simulink model "stereo_ibvs_core_backup_20260724_005942"  (R2025b)
settings: Solver=FixedStepDiscrete  StartTime=0.0  StopTime=10  FixedStep=cfg.Ts  RelTol=1e-3
InitFcn:
  | modelPath = get_param(bdroot,'FileName');
  |                                                                                       simulinkPath = fileparts(fileparts(modelPath));
  |                                                                                       configPath = fullfile(simulinkPath,'config','stereo_ibvs_config.m');
  |                                                                                       if ~isfile(configPath), error('StereoIBVS:ConfigNotFound','找不到配置文件：%s',configPath); end
  |                                                                                       run(configPath);
undefined symbols (not defined in the file): cfg
(part 2 of 4)

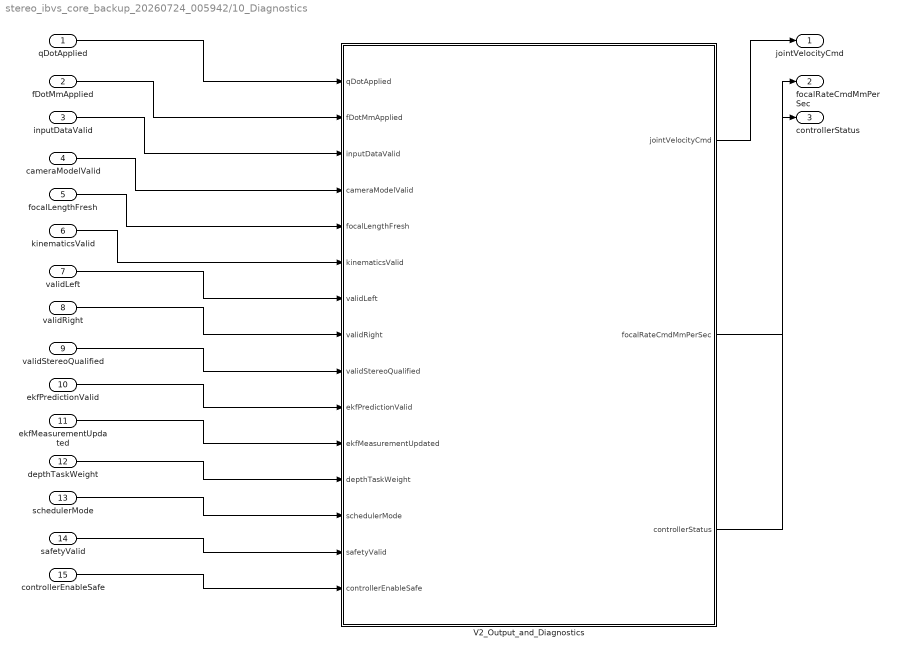
== system stereo_ibvs_core_backup_20260724_005942/10_Diagnostics ==
  qDotApplied : Inport  OutDataTypeStr=double  PortDimensions=[7 1]
  fDotMmApplied : Inport  Port=2  OutDataTypeStr=double  PortDimensions=[2 1]
  inputDataValid : Inport  Port=3  OutDataTypeStr=double  PortDimensions=1
  cameraModelValid : Inport  Port=4  OutDataTypeStr=double  PortDimensions=1
  focalLengthFresh : Inport  Port=5  OutDataTypeStr=double  PortDimensions=1
  kinematicsValid : Inport  Port=6  OutDataTypeStr=double  PortDimensions=1
  validLeft : Inport  Port=7  OutDataTypeStr=double  PortDimensions=1
  validRight : Inport  Port=8  OutDataTypeStr=double  PortDimensions=1
  validStereoQualified : Inport  Port=9  OutDataTypeStr=double  PortDimensions=1
  ekfPredictionValid : Inport  Port=10  OutDataTypeStr=double  PortDimensions=1
  ekfMeasurementUpdated : Inport  Port=11  OutDataTypeStr=double  PortDimensions=1
  depthTaskWeight : Inport  Port=12  OutDataTypeStr=double  PortDimensions=1
  schedulerMode : Inport  Port=13  OutDataTypeStr=double  PortDimensions=1
  safetyValid : Inport  Port=14  OutDataTypeStr=double  PortDimensions=1
  controllerEnableSafe : Inport  Port=15  OutDataTypeStr=double  PortDimensions=1
  V2_Output_and_Diagnostics : MATLAB Function  TreatAsAtomicUnit=on
  jointVelocityCmd : Outport  PortDimensions=[7 1]
  focalRateCmdMmPerSec : Outport  Port=2  PortDimensions=[2 1]
  controllerStatus : Outport  Port=3  PortDimensions=[13 1]
  wires:
  ? -> ?
  qDotApplied/1 -> V2_Output_and_Diagnostics/1(qDotApplied)
  fDotMmApplied/1 -> V2_Output_and_Diagnostics/2(fDotMmApplied)
  inputDataValid/1 -> V2_Output_and_Diagnostics/3(inputDataValid)
  cameraModelValid/1 -> V2_Output_and_Diagnostics/4(cameraModelValid)
  focalLengthFresh/1 -> V2_Output_and_Diagnostics/5(focalLengthFresh)
  kinematicsValid/1 -> V2_Output_and_Diagnostics/6(kinematicsValid)
  validLeft/1 -> V2_Output_and_Diagnostics/7(validLeft)
  validRight/1 -> V2_Output_and_Diagnostics/8(validRight)
  validStereoQualified/1 -> V2_Output_and_Diagnostics/9(validStereoQualified)
  ekfPredictionValid/1 -> V2_Output_and_Diagnostics/10(ekfPredictionValid)
  ekfMeasurementUpdated/1 -> V2_Output_and_Diagnostics/11(ekfMeasurementUpdated)
  depthTaskWeight/1 -> V2_Output_and_Diagnostics/12(depthTaskWeight)
  schedulerMode/1 -> V2_Output_and_Diagnostics/13(schedulerMode)
  safetyValid/1 -> V2_Output_and_Diagnostics/14(safetyValid)
  controllerEnableSafe/1 -> V2_Output_and_Diagnostics/15(controllerEnableSafe)
  V2_Output_and_Diagnostics/1(jointVelocityCmd) -> jointVelocityCmd/1
  V2_Output_and_Diagnostics/2(focalRateCmdMmPerSec) -> focalRateCmdMmPerSec/1
  V2_Output_and_Diagnostics/3(controllerStatus) -> controllerStatus/1

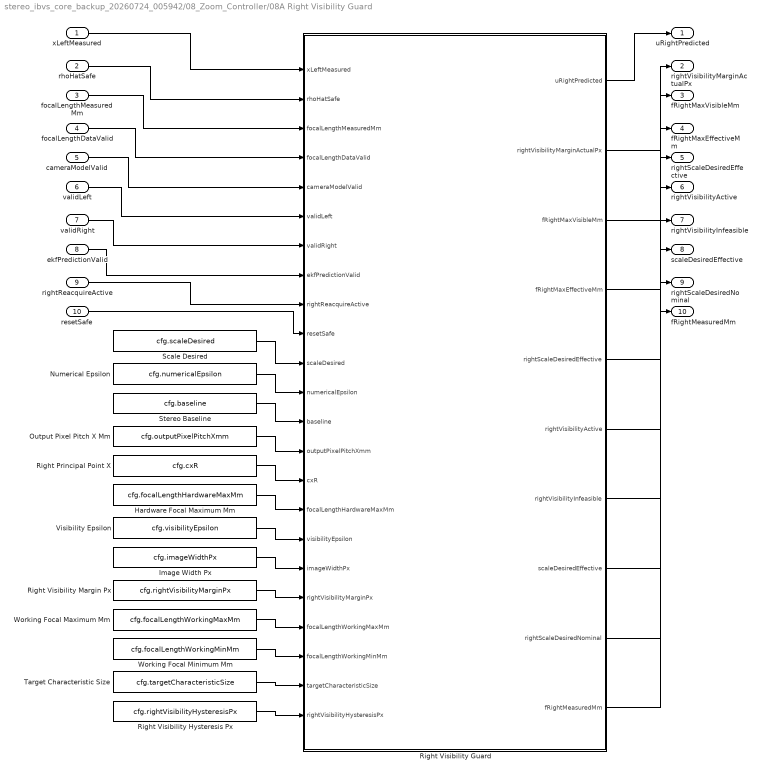
== system stereo_ibvs_core_backup_20260724_005942/08_Zoom_Controller/08A Right Visibility Guard ==
  xLeftMeasured : Inport  OutDataTypeStr=double  PortDimensions=1
  rhoHatSafe : Inport  Port=2  OutDataTypeStr=double  PortDimensions=1
  focalLengthMeasuredMm : Inport  Port=3  OutDataTypeStr=double  PortDimensions=[2 1]
  focalLengthDataValid : Inport  Port=4  OutDataTypeStr=double  PortDimensions=1
  cameraModelValid : Inport  Port=5  OutDataTypeStr=double  PortDimensions=1
  validLeft : Inport  Port=6  OutDataTypeStr=double  PortDimensions=1
  validRight : Inport  Port=7  OutDataTypeStr=double  PortDimensions=1
  ekfPredictionValid : Inport  Port=8  OutDataTypeStr=double  PortDimensions=1
  rightReacquireActive : Inport  Port=9  OutDataTypeStr=double  PortDimensions=1
  resetSafe : Inport  Port=10  OutDataTypeStr=double  PortDimensions=1
  Hardware Focal Maximum Mm : Constant  Value=cfg.focalLengthHardwareMaxMm  OutDataTypeStr=double  SampleTime=-1
  Image Width Px : Constant  Value=cfg.imageWidthPx  OutDataTypeStr=double  SampleTime=-1
  Numerical Epsilon : Constant  Value=cfg.numericalEpsilon  OutDataTypeStr=double  SampleTime=-1
  Output Pixel Pitch X Mm : Constant  Value=cfg.outputPixelPitchXmm  OutDataTypeStr=double  SampleTime=-1
  Right Principal Point X : Constant  Value=cfg.cxR  OutDataTypeStr=double  SampleTime=-1
  Right Visibility Guard : MATLAB Function  TreatAsAtomicUnit=on
  Right Visibility Hysteresis Px : Constant  Value=cfg.rightVisibilityHysteresisPx  OutDataTypeStr=double  SampleTime=-1
  Right Visibility Margin Px : Constant  Value=cfg.rightVisibilityMarginPx  OutDataTypeStr=double  SampleTime=-1
  Scale Desired : Constant  Value=cfg.scaleDesired  OutDataTypeStr=double  SampleTime=-1
  Stereo Baseline : Constant  Value=cfg.baseline  OutDataTypeStr=double  SampleTime=-1
  Target Characteristic Size : Constant  Value=cfg.targetCharacteristicSize  OutDataTypeStr=double  SampleTime=-1
  Visibility Epsilon : Constant  Value=cfg.visibilityEpsilon  OutDataTypeStr=double  SampleTime=-1
  Working Focal Maximum Mm : Constant  Value=cfg.focalLengthWorkingMaxMm  OutDataTypeStr=double  SampleTime=-1
  Working Focal Minimum Mm : Constant  Value=cfg.focalLengthWorkingMinMm  OutDataTypeStr=double  SampleTime=-1
  uRightPredicted : Outport  PortDimensions=1
  rightVisibilityMarginActualPx : Outport  Port=2  PortDimensions=1
  fRightMaxVisibleMm : Outport  Port=3  PortDimensions=1
  fRightMaxEffectiveMm : Outport  Port=4  PortDimensions=1
  rightScaleDesiredEffective : Outport  Port=5  PortDimensions=1
  rightVisibilityActive : Outport  Port=6  PortDimensions=1
  rightVisibilityInfeasible : Outport  Port=7  PortDimensions=1
  scaleDesiredEffective : Outport  Port=8  PortDimensions=[2 1]
  rightScaleDesiredNominal : Outport  Port=9  PortDimensions=1
  fRightMeasuredMm : Outport  Port=10  PortDimensions=1
  wires:
  ? -> ?
  xLeftMeasured/1 -> Right Visibility Guard/1(xLeftMeasured)
  rhoHatSafe/1 -> Right Visibility Guard/2(rhoHatSafe)
  focalLengthMeasuredMm/1 -> Right Visibility Guard/3(focalLengthMeasuredMm)
  focalLengthDataValid/1 -> Right Visibility Guard/4(focalLengthDataValid)
  cameraModelValid/1 -> Right Visibility Guard/5(cameraModelValid)
  validLeft/1 -> Right Visibility Guard/6(validLeft)
  validRight/1 -> Right Visibility Guard/7(validRight)
  ekfPredictionValid/1 -> Right Visibility Guard/8(ekfPredictionValid)
  rightReacquireActive/1 -> Right Visibility Guard/9(rightReacquireActive)
  resetSafe/1 -> Right Visibility Guard/10(resetSafe)
  Scale Desired/1 -> Right Visibility Guard/11(scaleDesired)
  Numerical Epsilon/1 -> Right Visibility Guard/12(numericalEpsilon)
  Stereo Baseline/1 -> Right Visibility Guard/13(baseline)
  Output Pixel Pitch X Mm/1 -> Right Visibility Guard/14(outputPixelPitchXmm)
  Right Principal Point X/1 -> Right Visibility Guard/15(cxR)
  Hardware Focal Maximum Mm/1 -> Right Visibility Guard/16(focalLengthHardwareMaxMm)
  Visibility Epsilon/1 -> Right Visibility Guard/17(visibilityEpsilon)
  Image Width Px/1 -> Right Visibility Guard/18(imageWidthPx)
  Right Visibility Margin Px/1 -> Right Visibility Guard/19(rightVisibilityMarginPx)
  Working Focal Maximum Mm/1 -> Right Visibility Guard/20(focalLengthWorkingMaxMm)
  Working Focal Minimum Mm/1 -> Right Visibility Guard/21(focalLengthWorkingMinMm)
  Target Characteristic Size/1 -> Right Visibility Guard/22(targetCharacteristicSize)
  Right Visibility Hysteresis Px/1 -> Right Visibility Guard/23(rightVisibilityHysteresisPx)
  Right Visibility Guard/1(uRightPredicted) -> uRightPredicted/1
  Right Visibility Guard/2(rightVisibilityMarginActualPx) -> rightVisibilityMarginActualPx/1
  Right Visibility Guard/3(fRightMaxVisibleMm) -> fRightMaxVisibleMm/1
  Right Visibility Guard/4(fRightMaxEffectiveMm) -> fRightMaxEffectiveMm/1
  Right Visibility Guard/5(rightScaleDesiredEffective) -> rightScaleDesiredEffective/1
  Right Visibility Guard/6(rightVisibilityActive) -> rightVisibilityActive/1
  Right Visibility Guard/7(rightVisibilityInfeasible) -> rightVisibilityInfeasible/1
  Right Visibility Guard/8(scaleDesiredEffective) -> scaleDesiredEffective/1
  Right Visibility Guard/9(rightScaleDesiredNominal) -> rightScaleDesiredNominal/1
  Right Visibility Guard/10(fRightMeasuredMm) -> fRightMeasuredMm/1

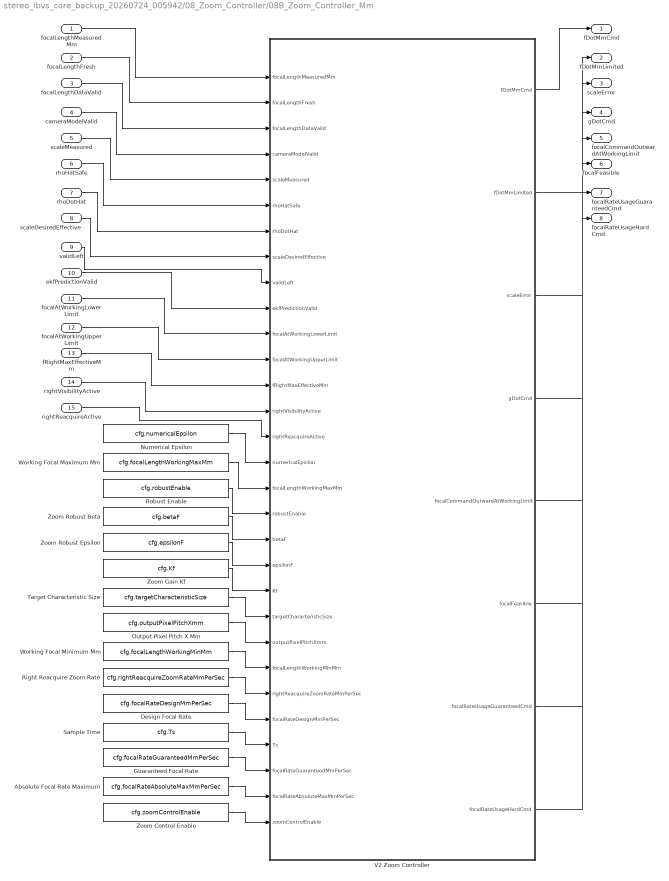
== system stereo_ibvs_core_backup_20260724_005942/08_Zoom_Controller/08B_Zoom_Controller_Mm ==
  focalLengthMeasuredMm : Inport  OutDataTypeStr=double  PortDimensions=[2 1]
  focalLengthFresh : Inport  Port=2  OutDataTypeStr=double  PortDimensions=1
  focalLengthDataValid : Inport  Port=3  OutDataTypeStr=double  PortDimensions=1
  cameraModelValid : Inport  Port=4  OutDataTypeStr=double  PortDimensions=1
  scaleMeasured : Inport  Port=5  OutDataTypeStr=double  PortDimensions=[2 1]
  rhoHatSafe : Inport  Port=6  OutDataTypeStr=double  PortDimensions=1
  rhoDotHat : Inport  Port=7  OutDataTypeStr=double  PortDimensions=[2 1]
  scaleDesiredEffective : Inport  Port=8  OutDataTypeStr=double  PortDimensions=[2 1]
  validLeft : Inport  Port=9  OutDataTypeStr=double  PortDimensions=1
  ekfPredictionValid : Inport  Port=10  OutDataTypeStr=double  PortDimensions=1
  focalAtWorkingLowerLimit : Inport  Port=11  OutDataTypeStr=double  PortDimensions=[2 1]
  focalAtWorkingUpperLimit : Inport  Port=12  OutDataTypeStr=double  PortDimensions=[2 1]
  fRightMaxEffectiveMm : Inport  Port=13  OutDataTypeStr=double  PortDimensions=1
  rightVisibilityActive : Inport  Port=14  OutDataTypeStr=double  PortDimensions=1
  rightReacquireActive : Inport  Port=15  OutDataTypeStr=double  PortDimensions=1
  Absolute Focal Rate Maximum : Constant  Value=cfg.focalRateAbsoluteMaxMmPerSec  OutDataTypeStr=double  SampleTime=-1
  Design Focal Rate : Constant  Value=cfg.focalRateDesignMmPerSec  OutDataTypeStr=double  SampleTime=-1
  Guaranteed Focal Rate : Constant  Value=cfg.focalRateGuaranteedMmPerSec  OutDataTypeStr=double  SampleTime=-1
  Numerical Epsilon : Constant  Value=cfg.numericalEpsilon  OutDataTypeStr=double  SampleTime=-1
  Output Pixel Pitch X Mm : Constant  Value=cfg.outputPixelPitchXmm  OutDataTypeStr=double  SampleTime=-1
  Right Reacquire Zoom Rate : Constant  Value=cfg.rightReacquireZoomRateMmPerSec  OutDataTypeStr=double  SampleTime=-1
  Robust Enable : Constant  Value=cfg.robustEnable  OutDataTypeStr=double  SampleTime=-1
  Sample Time : Constant  Value=cfg.Ts  OutDataTypeStr=double  SampleTime=-1
  Target Characteristic Size : Constant  Value=cfg.targetCharacteristicSize  OutDataTypeStr=double  SampleTime=-1
  V2 Zoom Controller : MATLAB Function  TreatAsAtomicUnit=on
  Working Focal Maximum Mm : Constant  Value=cfg.focalLengthWorkingMaxMm  OutDataTypeStr=double  SampleTime=-1
  Working Focal Minimum Mm : Constant  Value=cfg.focalLengthWorkingMinMm  OutDataTypeStr=double  SampleTime=-1
  Zoom Control Enable : Constant  Value=cfg.zoomControlEnable  OutDataTypeStr=double  SampleTime=-1
  Zoom Gain Kf : Constant  Value=cfg.Kf  OutDataTypeStr=double  SampleTime=-1
  Zoom Robust Beta : Constant  Value=cfg.betaF  OutDataTypeStr=double  SampleTime=-1
  Zoom Robust Epsilon : Constant  Value=cfg.epsilonF  OutDataTypeStr=double  SampleTime=-1
  fDotMmCmd : Outport  PortDimensions=[2 1]
  fDotMmLimited : Outport  Port=2  PortDimensions=[2 1]
  scaleError : Outport  Port=3  PortDimensions=[2 1]
  gDotCmd : Outport  Port=4  PortDimensions=[2 1]
  focalCommandOutwardAtWorkingLimit : Outport  Port=5  PortDimensions=[2 1]
  focalFeasible : Outport  Port=6  PortDimensions=[2 1]
  focalRateUsageGuaranteedCmd : Outport  Port=7  PortDimensions=[2 1]
  focalRateUsageHardCmd : Outport  Port=8  PortDimensions=[2 1]
  wires:
  ? -> ?
  focalLengthMeasuredMm/1 -> V2 Zoom Controller/1(focalLengthMeasuredMm)
  focalLengthFresh/1 -> V2 Zoom Controller/2(focalLengthFresh)
  focalLengthDataValid/1 -> V2 Zoom Controller/3(focalLengthDataValid)
  cameraModelValid/1 -> V2 Zoom Controller/4(cameraModelValid)
  scaleMeasured/1 -> V2 Zoom Controller/5(scaleMeasured)
  rhoHatSafe/1 -> V2 Zoom Controller/6(rhoHatSafe)
  rhoDotHat/1 -> V2 Zoom Controller/7(rhoDotHat)
  scaleDesiredEffective/1 -> V2 Zoom Controller/8(scaleDesiredEffective)
  validLeft/1 -> V2 Zoom Controller/9(validLeft)
  ekfPredictionValid/1 -> V2 Zoom Controller/10(ekfPredictionValid)
  focalAtWorkingLowerLimit/1 -> V2 Zoom Controller/11(focalAtWorkingLowerLimit)
  focalAtWorkingUpperLimit/1 -> V2 Zoom Controller/12(focalAtWorkingUpperLimit)
  fRightMaxEffectiveMm/1 -> V2 Zoom Controller/13(fRightMaxEffectiveMm)
  rightVisibilityActive/1 -> V2 Zoom Controller/14(rightVisibilityActive)
  rightReacquireActive/1 -> V2 Zoom Controller/15(rightReacquireActive)
  Numerical Epsilon/1 -> V2 Zoom Controller/16(numericalEpsilon)
  Working Focal Maximum Mm/1 -> V2 Zoom Controller/17(focalLengthWorkingMaxMm)
  Robust Enable/1 -> V2 Zoom Controller/18(robustEnable)
  Zoom Robust Beta/1 -> V2 Zoom Controller/19(betaF)
  Zoom Robust Epsilon/1 -> V2 Zoom Controller/20(epsilonF)
  Zoom Gain Kf/1 -> V2 Zoom Controller/21(Kf)
  Target Characteristic Size/1 -> V2 Zoom Controller/22(targetCharacteristicSize)
  Output Pixel Pitch X Mm/1 -> V2 Zoom Controller/23(outputPixelPitchXmm)
  Working Focal Minimum Mm/1 -> V2 Zoom Controller/24(focalLengthWorkingMinMm)
  Right Reacquire Zoom Rate/1 -> V2 Zoom Controller/25(rightReacquireZoomRateMmPerSec)
  Design Focal Rate/1 -> V2 Zoom Controller/26(focalRateDesignMmPerSec)
  Sample Time/1 -> V2 Zoom Controller/27(Ts)
  Guaranteed Focal Rate/1 -> V2 Zoom Controller/28(focalRateGuaranteedMmPerSec)
  Absolute Focal Rate Maximum/1 -> V2 Zoom Controller/29(focalRateAbsoluteMaxMmPerSec)
  Zoom Control Enable/1 -> V2 Zoom Controller/30(zoomControlEnable)
  V2 Zoom Controller/1(fDotMmCmd) -> fDotMmCmd/1
  V2 Zoom Controller/2(fDotMmLimited) -> fDotMmLimited/1
  V2 Zoom Controller/3(scaleError) -> scaleError/1
  V2 Zoom Controller/4(gDotCmd) -> gDotCmd/1
  V2 Zoom Controller/5(focalCommandOutwardAtWorkingLimit) -> focalCommandOutwardAtWorkingLimit/1
  V2 Zoom Controller/6(focalFeasible) -> focalFeasible/1
  V2 Zoom Controller/7(focalRateUsageGuaranteedCmd) -> focalRateUsageGuaranteedCmd/1
  V2 Zoom Controller/8(focalRateUsageHardCmd) -> focalRateUsageHardCmd/1

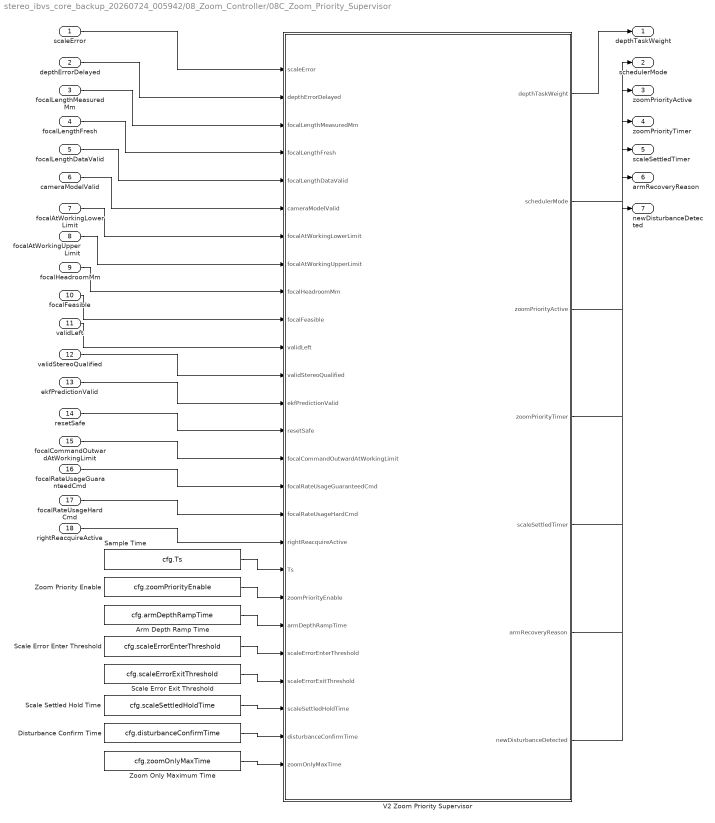
== system stereo_ibvs_core_backup_20260724_005942/08_Zoom_Controller/08C_Zoom_Priority_Supervisor ==
  scaleError : Inport  OutDataTypeStr=double  PortDimensions=[2 1]
  depthErrorDelayed : Inport  Port=2  OutDataTypeStr=double  PortDimensions=1
  focalLengthMeasuredMm : Inport  Port=3  OutDataTypeStr=double  PortDimensions=[2 1]
  focalLengthFresh : Inport  Port=4  OutDataTypeStr=double  PortDimensions=1
  focalLengthDataValid : Inport  Port=5  OutDataTypeStr=double  PortDimensions=1
  cameraModelValid : Inport  Port=6  OutDataTypeStr=double  PortDimensions=1
  focalAtWorkingLowerLimit : Inport  Port=7  OutDataTypeStr=double  PortDimensions=[2 1]
  focalAtWorkingUpperLimit : Inport  Port=8  OutDataTypeStr=double  PortDimensions=[2 1]
  focalHeadroomMm : Inport  Port=9  OutDataTypeStr=double  PortDimensions=[2 1]
  focalFeasible : Inport  Port=10  OutDataTypeStr=double  PortDimensions=[2 1]
  validLeft : Inport  Port=11  OutDataTypeStr=double  PortDimensions=1
  validStereoQualified : Inport  Port=12  OutDataTypeStr=double  PortDimensions=1
  ekfPredictionValid : Inport  Port=13  OutDataTypeStr=double  PortDimensions=1
  resetSafe : Inport  Port=14  OutDataTypeStr=double  PortDimensions=1
  focalCommandOutwardAtWorkingLimit : Inport  Port=15  OutDataTypeStr=double  PortDimensions=[2 1]
  focalRateUsageGuaranteedCmd : Inport  Port=16  OutDataTypeStr=double  PortDimensions=[2 1]
  focalRateUsageHardCmd : Inport  Port=17  OutDataTypeStr=double  PortDimensions=[2 1]
  rightReacquireActive : Inport  Port=18  OutDataTypeStr=double  PortDimensions=1
  Arm Depth Ramp Time : Constant  Value=cfg.armDepthRampTime  OutDataTypeStr=double  SampleTime=-1
  Disturbance Confirm Time : Constant  Value=cfg.disturbanceConfirmTime  OutDataTypeStr=double  SampleTime=-1
  Sample Time : Constant  Value=cfg.Ts  OutDataTypeStr=double  SampleTime=-1
  Scale Error Enter Threshold : Constant  Value=cfg.scaleErrorEnterThreshold  OutDataTypeStr=double  SampleTime=-1
  Scale Error Exit Threshold : Constant  Value=cfg.scaleErrorExitThreshold  OutDataTypeStr=double  SampleTime=-1
  Scale Settled Hold Time : Constant  Value=cfg.scaleSettledHoldTime  OutDataTypeStr=double  SampleTime=-1
  V2 Zoom Priority Supervisor : MATLAB Function  TreatAsAtomicUnit=on
  Zoom Only Maximum Time : Constant  Value=cfg.zoomOnlyMaxTime  OutDataTypeStr=double  SampleTime=-1
  Zoom Priority Enable : Constant  Value=cfg.zoomPriorityEnable  OutDataTypeStr=double  SampleTime=-1
  depthTaskWeight : Outport  PortDimensions=1
  schedulerMode : Outport  Port=2  PortDimensions=1
  zoomPriorityActive : Outport  Port=3  PortDimensions=1
  zoomPriorityTimer : Outport  Port=4  PortDimensions=1
  scaleSettledTimer : Outport  Port=5  PortDimensions=1
  armRecoveryReason : Outport  Port=6  PortDimensions=1
  newDisturbanceDetected : Outport  Port=7  PortDimensions=1
  wires:
  ? -> ?
  scaleError/1 -> V2 Zoom Priority Supervisor/1(scaleError)
  depthErrorDelayed/1 -> V2 Zoom Priority Supervisor/2(depthErrorDelayed)
  focalLengthMeasuredMm/1 -> V2 Zoom Priority Supervisor/3(focalLengthMeasuredMm)
  focalLengthFresh/1 -> V2 Zoom Priority Supervisor/4(focalLengthFresh)
  focalLengthDataValid/1 -> V2 Zoom Priority Supervisor/5(focalLengthDataValid)
  cameraModelValid/1 -> V2 Zoom Priority Supervisor/6(cameraModelValid)
  focalAtWorkingLowerLimit/1 -> V2 Zoom Priority Supervisor/7(focalAtWorkingLowerLimit)
  focalAtWorkingUpperLimit/1 -> V2 Zoom Priority Supervisor/8(focalAtWorkingUpperLimit)
  focalHeadroomMm/1 -> V2 Zoom Priority Supervisor/9(focalHeadroomMm)
  focalFeasible/1 -> V2 Zoom Priority Supervisor/10(focalFeasible)
  validLeft/1 -> V2 Zoom Priority Supervisor/11(validLeft)
  validStereoQualified/1 -> V2 Zoom Priority Supervisor/12(validStereoQualified)
  ekfPredictionValid/1 -> V2 Zoom Priority Supervisor/13(ekfPredictionValid)
  resetSafe/1 -> V2 Zoom Priority Supervisor/14(resetSafe)
  focalCommandOutwardAtWorkingLimit/1 -> V2 Zoom Priority Supervisor/15(focalCommandOutwardAtWorkingLimit)
  focalRateUsageGuaranteedCmd/1 -> V2 Zoom Priority Supervisor/16(focalRateUsageGuaranteedCmd)
  focalRateUsageHardCmd/1 -> V2 Zoom Priority Supervisor/17(focalRateUsageHardCmd)
  rightReacquireActive/1 -> V2 Zoom Priority Supervisor/18(rightReacquireActive)
  Sample Time/1 -> V2 Zoom Priority Supervisor/19(Ts)
  Zoom Priority Enable/1 -> V2 Zoom Priority Supervisor/20(zoomPriorityEnable)
  Arm Depth Ramp Time/1 -> V2 Zoom Priority Supervisor/21(armDepthRampTime)
  Scale Error Enter Threshold/1 -> V2 Zoom Priority Supervisor/22(scaleErrorEnterThreshold)
  Scale Error Exit Threshold/1 -> V2 Zoom Priority Supervisor/23(scaleErrorExitThreshold)
  Scale Settled Hold Time/1 -> V2 Zoom Priority Supervisor/24(scaleSettledHoldTime)
  Disturbance Confirm Time/1 -> V2 Zoom Priority Supervisor/25(disturbanceConfirmTime)
  Zoom Only Maximum Time/1 -> V2 Zoom Priority Supervisor/26(zoomOnlyMaxTime)
  V2 Zoom Priority Supervisor/1(depthTaskWeight) -> depthTaskWeight/1
  V2 Zoom Priority Supervisor/2(schedulerMode) -> schedulerMode/1
  V2 Zoom Priority Supervisor/3(zoomPriorityActive) -> zoomPriorityActive/1
  V2 Zoom Priority Supervisor/4(zoomPriorityTimer) -> zoomPriorityTimer/1
  V2 Zoom Priority Supervisor/5(scaleSettledTimer) -> scaleSettledTimer/1
  V2 Zoom Priority Supervisor/6(armRecoveryReason) -> armRecoveryReason/1
  V2 Zoom Priority Supervisor/7(newDisturbanceDetected) -> newDisturbanceDetected/1

== matlab function stereo_ibvs_core_backup_20260724_005942/03_Feature_Processing/Normalize and Validate Features ==
  data: pixelMeasurement input; normalizedFeatureMeasured output; scaleMeasuredRaw input; fxMeasuredPx input; fyMeasuredPx input; validLeft input; validRight input; visionMeasurementNew input; resetSafe input; cfg_numericalEpsilon input; cfg_cxL input; cfg_cyL input; cfg_cxR input; cfg_cyR input; cfg_baseline input; cfg_disparityMin input; cfg_rhoMin input; cfg_rhoMax input; cfg_rightReacquireValidSamples input; cLMeasured output; cRMeasured output; scaleMeasured output; zMeasured output; xLeftMeasured output; yLeftMeasured output; xRightMeasured output; disparityNormalized output; rhoMeasured output; validDisparity output; stereoMeasurementEnable output; validStereoQualified output; rightReacquireActive output; rightReacquireCount output; uRightMeasured output
function [ ...
    normalizedFeatureMeasured, ...
    cLMeasured, ...
    cRMeasured, ...
    scaleMeasured, ...
    zMeasured, ...
    xLeftMeasured, ...
    yLeftMeasured, ...
    xRightMeasured, ...
    disparityNormalized, ...
    rhoMeasured, ...
    validDisparity, ...
    stereoMeasurementEnable, ...
    validStereoQualified, ...
    rightReacquireActive, ...
    rightReacquireCount, ...
    uRightMeasured] = fcn( ...
    pixelMeasurement, ...
    scaleMeasuredRaw, ...
    fxMeasuredPx, ...
    fyMeasuredPx, ...
    validLeft, ...
    validRight, ...
    visionMeasurementNew, ...
    resetSafe, ...
    cfg_numericalEpsilon, ...
    cfg_cxL, ...
    cfg_cyL, ...
    cfg_cxR, ...
    cfg_cyR, ...
    cfg_baseline, ...
    cfg_disparityMin, ...
    cfg_rhoMin, ...
    cfg_rhoMax, ...
    cfg_rightReacquireValidSamples)
%#codegen
% V2实机视觉测量提取与双目有效性管理。
% cfg_* 均由外部 Constant 块输入，不再登记为 MATLAB Function Parameter。

%% 固定尺寸输出
normalizedFeatureMeasured = zeros(4,1);
cLMeasured = zeros(2,1);
cRMeasured = zeros(2,1);
scaleMeasured = zeros(2,1);
zMeasured = zeros(3,1);

xLeftMeasured = 0;
yLeftMeasured = 0;
xRightMeasured = 0;
disparityNormalized = 0;
rhoMeasured = 0;

validDisparity = 0;
stereoMeasurementEnable = 0;
validStereoQualified = 0;
rightReacquireActive = 0;
rightReacquireCount = 0;
uRightMeasured = 0;

%% 右相机重捕获状态
persistent consecutiveValid reacquire

if isempty(consecutiveValid)
    consecutiveValid = 0.0;
    reacquire = 1.0;
end

%% 输入整理
pixels = reshape(pixelMeasurement,4,1);
scales = reshape(scaleMeasuredRaw,2,1);
fx = reshape(fxMeasuredPx,2,1);
fy = reshape(fyMeasuredPx,2,1);

leftValidFlag = ...
    isfinite(validLeft) && validLeft > 0.5;
rightValidFlag = ...
    isfinite(validRight) && validRight > 0.5;
newMeasurement = ...
    isfinite(visionMeasurementNew) && visionMeasurementNew > 0.5;
resetRequested = ...
    isfinite(resetSafe) && resetSafe > 0.5;

parameterFinite = all(isfinite([ ...
    cfg_numericalEpsilon
    cfg_cxL
    cfg_cyL
    cfg_cxR
    cfg_cyR
    cfg_baseline
    cfg_disparityMin
    cfg_rhoMin
    cfg_rhoMax
    cfg_rightReacquireValidSamples]));

parameterValid = ...
    parameterFinite && ...
    cfg_numericalEpsilon > 0 && ...
    cfg_baseline > cfg_numericalEpsilon && ...
    cfg_disparityMin >= 0 && ...
    cfg_rhoMin > 0 && ...
    cfg_rhoMax >= cfg_rhoMin && ...
    cfg_rightReacquireValidSamples >= 1;

reacquireRequired = 1.0;
if parameterValid
    reacquireRequired = max( ...
        1.0, ...
        floor(cfg_rightReacquireValidSamples));
end

geometryInputFinite = ...
    all(isfinite(pixels)) && ...
    all(isfinite(fx)) && ...
    all(isfinite(fy)) && ...
    parameterValid;

leftIntrinsicsValid = ...
    geometryInputFinite && ...
    fx(1) > cfg_numericalEpsilon && ...
    fy(1) > cfg_numericalEpsilon;

rightIntrinsicsValid = ...
    geometryInputFinite && ...
    fx(2) > cfg_numericalEpsilon && ...
    fy(2) > cfg_numericalEpsilon;

leftFeatureValid = ...
    leftValidFlag && leftIntrinsicsValid;
rightFeatureValid = ...
    rightValidFlag && rightIntrinsicsValid;

%% 像素坐标归一化
if leftFeatureValid
    cLMeasured = [ ...
        (pixels(1) - cfg_cxL) / fx(1)
        (pixels(2) - cfg_cyL) / fy(1)];
end

if rightFeatureValid
    cRMeasured = [ ...
        (pixels(3) - cfg_cxR) / fx(2)
        (pixels(4) - cfg_cyR) / fy(2)];

    % 只有右相机测量有效时才输出右相机像素位置。
    uRightMeasured = pixels(3);
end

% Scale无效时仅将对应Scale置零，不影响中心和双目几何计算。
if leftFeatureValid && ...
        isfinite(scales(1)) && scales(1) > 0
    scaleMeasured(1) = scales(1);
end

if rightFeatureValid && ...
        isfinite(scales(2)) && scales(2) > 0
    scaleMeasured(2) = scales(2);
end

normalizedFeatureMeasured = [cLMeasured; cRMeasured];

xLeftMeasured = cLMeasured(1);
yLeftMeasured = cLMeasured(2);
xRightMeasured = cRMeasured(1);

%% 双目视差与逆深度测量
if leftFeatureValid && rightFeatureValid
    disparityNormalized = ...
        xLeftMeasured - xRightMeasured;

    candidateRho = ...
        disparityNormalized / cfg_baseline;

    validDisparity = double( ...
        isfinite(candidateRho) && ...
        disparityNormalized > cfg_disparityMin && ...
        candidateRho >= cfg_rhoMin && ...
        candidateRho <= cfg_rhoMax);

    if validDisparity > 0.5
        rhoMeasured = candidateRho;
    end
end

zMeasured = [ ...
    xLeftMeasured
    yLeftMeasured
    rhoMeasured];

%% 完整有限值保护
measurementOutputsFinite = ...
    all(isfinite(normalizedFeatureMeasured)) && ...
    all(isfinite(cLMeasured)) && ...
    all(isfinite(cRMeasured)) && ...
    all(isfinite(scaleMeasured)) && ...
    all(isfinite(zMeasured)) && ...
    isfinite(xLeftMeasured) && ...
    isfinite(yLeftMeasured) && ...
    isfinite(xRightMeasured) && ...
    isfinite(disparityNormalized) && ...
    isfinite(rhoMeasured) && ...
    isfinite(validDisparity) && ...
    isfinite(uRightMeasured);

if ~measurementOutputsFinite
    normalizedFeatureMeasured = zeros(4,1);
    cLMeasured = zeros(2,1);
    cRMeasured = zeros(2,1);
    scaleMeasured = zeros(2,1);
    zMeasured = zeros(3,1);

    xLeftMeasured = 0;
    yLeftMeasured = 0;
    xRightMeasured = 0;
    disparityNormalized = 0;
    rhoMeasured = 0;
    validDisparity = 0;
    uRightMeasured = 0;
end

%% 双目资格与右相机重捕获管理
rawStereoValid = ...
    measurementOutputsFinite && ...
    leftFeatureValid && ...
    rightFeatureValid && ...
    validDisparity > 0.5;

if resetRequested
    consecutiveValid = 0.0;
    reacquire = 1.0;

elseif newMeasurement
    if rawStereoValid
        consecutiveValid = min( ...
            consecutiveValid + 1.0, ...
            reacquireRequired);
    else
        consecutiveValid = 0.0;
    end

    if ~rawStereoValid
        reacquire = 1.0;
    elseif consecutiveValid >= reacquireRequired
        reacquire = 0.0;
    end
end

validStereoQualified = double( ...
    rawStereoValid && ...
    consecutiveValid >= reacquireRequired);

% 每个新视觉测量最多触发一次EKF校正。
stereoMeasurementEnable = double( ...
    newMeasurement && ...
    validStereoQualified > 0.5 && ...
    ~resetRequested);

rightReacquireActive = double( ...
    leftFeatureValid && ...
    reacquire > 0.5);

rightReacquireCount = consecutiveValid;
end

== matlab function stereo_ibvs_core_backup_20260724_005942/04_FR3_Camera_Kinematics/FR3 Camera Kinematics ==
  data: q input; pWCL output; cfg_T_W_B input; cfg_fr3OriginXYZ input; cfg_fr3OriginRPY input; cfg_fr3Axis input; cfg_fr3Joint8OriginXYZ input; cfg_fr3Joint8OriginRPY input; cfg_T_link8_CL input; cfg_T_CL_CR input; cfg_numericalEpsilon input; RWCL output; pWCR output; RWCR output; JL output; JR output; rankJL output; rcondJL output; rotationOrthogonalityError output; baselineLength output; baselineError output; stereoRotationError output; pWLink8 output; RWLink8 output; kinematicsValid output
function [ ...
    pWCL, ...
    RWCL, ...
    pWCR, ...
    RWCR, ...
    JL, ...
    JR, ...
    rankJL, ...
    rcondJL, ...
    rotationOrthogonalityError, ...
    baselineLength, ...
    baselineError, ...
    stereoRotationError, ...
    pWLink8, ...
    RWLink8, ...
    kinematicsValid] = fcn( ...
    q, ...
    cfg_T_W_B, ...
    cfg_fr3OriginXYZ, ...
    cfg_fr3OriginRPY, ...
    cfg_fr3Axis, ...
    cfg_fr3Joint8OriginXYZ, ...
    cfg_fr3Joint8OriginRPY, ...
    cfg_T_link8_CL, ...
    cfg_T_CL_CR, ...
    cfg_numericalEpsilon)
%#codegen
% V2 FR3双目相机运动学与诊断。

% 固定尺寸输出
pWCL = zeros(3,1);
RWCL = eye(3);
pWCR = zeros(3,1);
RWCR = eye(3);
JL = zeros(6,7);
JR = zeros(6,7);
rankJL = 0;
rcondJL = 0;
rotationOrthogonalityError = 0;
baselineLength = 0;
baselineError = 0;
stereoRotationError = 0;
pWLink8 = zeros(3,1);
RWLink8 = eye(3);
kinematicsValid = false;

% 输入整理和检查
qSafe = reshape(q,7,1);

inputValid = ...
    all(isfinite(qSafe)) && ...
    all(isfinite(cfg_T_W_B(:))) && ...
    all(isfinite(cfg_fr3OriginXYZ(:))) && ...
    all(isfinite(cfg_fr3OriginRPY(:))) && ...
    all(isfinite(cfg_fr3Axis(:))) && ...
    all(isfinite(cfg_fr3Joint8OriginXYZ(:))) && ...
    all(isfinite(cfg_fr3Joint8OriginRPY(:))) && ...
    all(isfinite(cfg_T_link8_CL(:))) && ...
    all(isfinite(cfg_T_CL_CR(:))) && ...
    isfinite(cfg_numericalEpsilon) && ...
    cfg_numericalEpsilon > 0;

if ~inputValid
    return;
end

% FR3正运动学
T = reshape(cfg_T_W_B,4,4);
jointOriginsW = zeros(3,7);
jointAxesW = zeros(3,7);

for jointIndex = 1:7
    T = T * makeTransform( ...
        cfg_fr3OriginXYZ(:,jointIndex), ...
        cfg_fr3OriginRPY(:,jointIndex));

    jointOriginsW(:,jointIndex) = T(1:3,4);

    axisLocal = cfg_fr3Axis(:,jointIndex);
    axisNorm = norm(axisLocal);

    if ~isfinite(axisNorm) || ...
            axisNorm <= cfg_numericalEpsilon
        return;
    end

    jointAxesW(:,jointIndex) = ...
        T(1:3,1:3) * axisLocal;

    T = T * axisRotation(axisLocal,qSafe(jointIndex));
end

% link8固定变换
T_W_link8 = T * makeTransform( ...
    cfg_fr3Joint8OriginXYZ, ...
    cfg_fr3Joint8OriginRPY);

pWLink8 = T_W_link8(1:3,4);
RWLink8 = T_W_link8(1:3,1:3);

% 左右相机位姿
T_W_CL = T_W_link8 * reshape(cfg_T_link8_CL,4,4);
T_W_CR = T_W_CL * reshape(cfg_T_CL_CR,4,4);

pWCL = T_W_CL(1:3,4);
RWCL = T_W_CL(1:3,1:3);
pWCR = T_W_CR(1:3,4);
RWCR = T_W_CR(1:3,1:3);

% 左相机光心的世界坐标Jacobian
JWLeft = zeros(6,7);

for jointIndex = 1:7
    JWLeft(1:3,jointIndex) = cross( ...
        jointAxesW(:,jointIndex), ...
        pWCL-jointOriginsW(:,jointIndex));

    JWLeft(4:6,jointIndex) = ...
        jointAxesW(:,jointIndex);
end

% 转换到左相机坐标系
R_CL_W = RWCL';

JL = [ ...
    R_CL_W, zeros(3,3)
    zeros(3,3), R_CL_W
    ] * JWLeft;

% 从左相机Jacobian转换到右相机坐标系
R_CL_CR = cfg_T_CL_CR(1:3,1:3);
p_CL_CR = cfg_T_CL_CR(1:3,4);

JR = [ ...
    R_CL_CR', -R_CL_CR'*skew3(p_CL_CR)
    zeros(3,3), R_CL_CR'
    ] * JL;

% 有限值检查
finiteResult = ...
    all(isfinite(pWCL)) && ...
    all(isfinite(RWCL(:))) && ...
    all(isfinite(pWCR)) && ...
    all(isfinite(RWCR(:))) && ...
    all(isfinite(JL(:))) && ...
    all(isfinite(JR(:))) && ...
    all(isfinite(pWLink8)) && ...
    all(isfinite(RWLink8(:)));

if ~finiteResult
    pWCL = zeros(3,1);
    RWCL = eye(3);
    pWCR = zeros(3,1);
    RWCR = eye(3);
    JL = zeros(6,7);
    JR = zeros(6,7);
    pWLink8 = zeros(3,1);
    RWLink8 = eye(3);
    return;
end

% V2运动学诊断
rankJL = rank(JL);
rcondJL = rcond(JL*JL');

rotationOrthogonalityError = max([ ...
    norm(RWCL'*RWCL-eye(3),'fro'), ...
    norm(RWCR'*RWCR-eye(3),'fro'), ...
    norm(RWLink8'*RWLink8-eye(3),'fro')]);

baselineLength = norm(pWCR-pWCL);
baselineError = abs( ...
    baselineLength-norm(p_CL_CR));

stereoRotationError = norm( ...
    RWCR-RWCL*R_CL_CR, ...
    'fro');

% 最终有效性判断
rotationTolerance = max( ...
    1e-6, ...
    100*cfg_numericalEpsilon);

diagnosticsFinite = ...
    isfinite(rankJL) && ...
    isfinite(rcondJL) && ...
    isfinite(rotationOrthogonalityError) && ...
    isfinite(baselineLength) && ...
    isfinite(baselineError) && ...
    isfinite(stereoRotationError);

rotationValid = ...
    rotationOrthogonalityError <= rotationTolerance && ...
    abs(det(RWCL)-1) <= rotationTolerance && ...
    abs(det(RWCR)-1) <= rotationTolerance && ...
    abs(det(RWLink8)-1) <= rotationTolerance;

kinematicsValid = ...
    diagnosticsFinite && ...
    rotationValid;

if ~kinematicsValid
    return;
end
end


function T = makeTransform(xyz,rpy)
T = eye(4);
T(1:3,1:3) = ...
    rotz3(rpy(3)) * ...
    roty3(rpy(2)) * ...
    rotx3(rpy(1));
T(1:3,4) = xyz;
end


function T = axisRotation(axis,q)
axisNorm = norm(axis);
unitAxis = axis / axisNorm;
K = skew3(unitAxis);
R = eye(3) + ...
    sin(q)*K + ...
    (1-cos(q))*(K*K);
T = eye(4);
T(1:3,1:3) = R;
end


function R = rotx3(angle)
c = cos(angle);
s = sin(angle);
R = [ ...
    1, 0, 0
    0, c, -s
    0, s, c
    ];
end


function R = roty3(angle)
c = cos(angle);
s = sin(angle);
R = [ ...
    c, 0, s
    0, 1, 0
    -s, 0, c
    ];
end


function R = rotz3(angle)
c = cos(angle);
s = sin(angle);
R = [ ...
    c, -s, 0
    s, c, 0
    0, 0, 1
    ];
end


function S = skew3(vector)
S = [ ...
    0, -vector(3), vector(2)
    vector(3), 0, -vector(1)
    -vector(2), vector(1), 0
    ];
end

== matlab function stereo_ibvs_core_backup_20260724_005942/05_Target_EKF/V2 Target EKF ==
  data: zMeasured input; pHatW output; measurementEnable input; visionMeasurementNewSafe input; pWCL input; RWCL input; fxMeasuredPx input; fyMeasuredPx input; resetSafe input; cfg_ekfX0 input; cfg_ekfP0 input; cfg_Ts input; cfg_sigmaJerk input; cfg_visibilityZMin input; cfg_numericalEpsilon input; cfg_rhoMin input; cfg_rhoMax input; cfg_pixelNoiseStd input; cfg_baseline input; cfg_ekfCovarianceJitter input; cfg_ekfSConditionMin input; cfg_ekfInitializationMode input; cfg_ekfRequireNewMeasurement input; vHatW output; aHatW output; pHatLeft output; vHatLeft output; rhoHatRaw output; rhoHatSafe output; innovation output; rhoInnovation output; innovationNorm output; traceP output; ekfPredictionValid output; ekfMeasurementUpdated output; ekfStateFinite output; minEigenvalueP output; symmetryErrorP output
function [ ...
    pHatW, ...
    vHatW, ...
    aHatW, ...
    pHatLeft, ...
    vHatLeft, ...
    rhoHatRaw, ...
    rhoHatSafe, ...
    innovation, ...
    rhoInnovation, ...
    innovationNorm, ...
    traceP, ...
    ekfPredictionValid, ...
    ekfMeasurementUpdated, ...
    ekfStateFinite, ...
    minEigenvalueP, ...
    symmetryErrorP] = fcn( ...
    zMeasured, ...
    measurementEnable, ...
    visionMeasurementNewSafe, ...
    pWCL, ...
    RWCL, ...
    fxMeasuredPx, ...
    fyMeasuredPx, ...
    resetSafe, ...
    cfg_ekfX0, ...
    cfg_ekfP0, ...
    cfg_Ts, ...
    cfg_sigmaJerk, ...
    cfg_visibilityZMin, ...
    cfg_numericalEpsilon, ...
    cfg_rhoMin, ...
    cfg_rhoMax, ...
    cfg_pixelNoiseStd, ...
    cfg_baseline, ...
    cfg_ekfCovarianceJitter, ...
    cfg_ekfSConditionMin, ...
    cfg_ekfInitializationMode, ...
    cfg_ekfRequireNewMeasurement)
%#codegen
% V2九状态世界坐标恒加速度EKF。
% 首次有效双目测量可直接初始化目标世界坐标位置。

% 固定尺寸输出
pHatW = zeros(3,1);
vHatW = zeros(3,1);
aHatW = zeros(3,1);
pHatLeft = zeros(3,1);
vHatLeft = zeros(3,1);
rhoHatRaw = 0;
rhoHatSafe = 0;
innovation = zeros(3,1);
rhoInnovation = 0;
innovationNorm = 0;
traceP = 0;
ekfPredictionValid = 0;
ekfMeasurementUpdated = 0;
ekfStateFinite = 0;
minEigenvalueP = 0;
symmetryErrorP = 0;

% 输入整理
z = reshape(zMeasured,3,1);
pCameraW = reshape(pWCL,3,1);
rotationCameraToWorld = reshape(RWCL,3,3);
fx = reshape(fxMeasuredPx,2,1);
fy = reshape(fyMeasuredPx,2,1);
ekfX0 = reshape(cfg_ekfX0,9,1);
ekfP0 = reshape(cfg_ekfP0,9,9);

% 持久状态
persistent x P initialized

if isempty(x)
    x = zeros(9,1);
    P = eye(9);
    initialized = false;
end

% 配置和输入有效性
configurationValid = ...
    all(isfinite(ekfX0)) && ...
    all(isfinite(ekfP0(:))) && ...
    isfinite(cfg_Ts) && cfg_Ts > 0 && ...
    isfinite(cfg_sigmaJerk) && cfg_sigmaJerk >= 0 && ...
    isfinite(cfg_visibilityZMin) && cfg_visibilityZMin > 0 && ...
    isfinite(cfg_numericalEpsilon) && cfg_numericalEpsilon > 0 && ...
    isfinite(cfg_rhoMin) && ...
    isfinite(cfg_rhoMax) && ...
    cfg_rhoMax > cfg_rhoMin && ...
    isfinite(cfg_pixelNoiseStd) && cfg_pixelNoiseStd >= 0 && ...
    isfinite(cfg_baseline) && ...
    cfg_baseline > cfg_numericalEpsilon && ...
    isfinite(cfg_ekfCovarianceJitter) && ...
    cfg_ekfCovarianceJitter >= 0 && ...
    isfinite(cfg_ekfSConditionMin) && ...
    cfg_ekfSConditionMin >= 0 && ...
    isfinite(cfg_ekfInitializationMode) && ...
    isfinite(cfg_ekfRequireNewMeasurement);

kinematicInputFinite = ...
    all(isfinite(pCameraW)) && ...
    all(isfinite(rotationCameraToWorld(:)));

focalPixelsValid = ...
    all(isfinite(fx)) && ...
    all(isfinite(fy)) && ...
    all(fx > cfg_numericalEpsilon) && ...
    all(fy > cfg_numericalEpsilon);

measurementEnableValid = ...
    isfinite(measurementEnable) && ...
    measurementEnable > 0.5;

visionNewValid = ...
    isfinite(visionMeasurementNewSafe) && ...
    visionMeasurementNewSafe > 0.5;

newMeasurementAccepted = ...
    cfg_ekfRequireNewMeasurement <= 0.5 || ...
    visionNewValid;

measurementFinite = all(isfinite(z));
measurementRhoValid = ...
    measurementFinite && ...
    z(3) >= cfg_rhoMin && ...
    z(3) <= cfg_rhoMax;

measurementAvailable = ...
    configurationValid && ...
    measurementEnableValid && ...
    newMeasurementAccepted && ...
    kinematicInputFinite && ...
    focalPixelsValid && ...
    measurementRhoValid;

resetRequested = ...
    isfinite(resetSafe) && ...
    resetSafe > 0.5;

if ~configurationValid
    initialized = false;
    return;
end

if resetRequested
    x = ekfX0;
    P = ekfP0;
    initialized = false;
    return;
end

% 固定初值模式兼容
fixedInitializationMode = ...
    cfg_ekfInitializationMode <= 0.5;

if ~initialized && fixedInitializationMode
    x = ekfX0;
    P = ekfP0;
    initialized = true;
end

% 首次有效双目测量初始化
justInitialized = false;

if ~initialized && measurementAvailable
    rhoInitial = z(3);
    depthInitial = 1/rhoInitial;

    pInitialLeft = [ ...
        z(1)*depthInitial
        z(2)*depthInitial
        depthInitial
    ];

    pInitialW = ...
        pCameraW + ...
        rotationCameraToWorld*pInitialLeft;

    initializationFinite = ...
        all(isfinite(pInitialLeft)) && ...
        all(isfinite(pInitialW)) && ...
        depthInitial > cfg_visibilityZMin;

    if initializationFinite
        x = [ ...
            pInitialW
            zeros(3,1)
            zeros(3,1)
        ];
        P = ekfP0;
        initialized = true;
        justInitialized = true;
        ekfMeasurementUpdated = 1;
    end
end

% 尚未初始化时保持安全无效输出
if ~initialized
    traceP = trace(0.5*(P+P'));
    return;
end

% 初始化当周期不重复执行预测和测量更新
if justInitialized
    pHatW = x(1:3);
    vHatW = x(4:6);
    aHatW = x(7:9);
    pHatLeft = ...
        rotationCameraToWorld' * ...
        (pHatW-pCameraW);
    vHatLeft = rotationCameraToWorld'*vHatW;

    ekfStateFinite = double( ...
        all(isfinite(x)) && ...
        all(isfinite(P(:))) && ...
        all(isfinite(pHatLeft)) && ...
        all(isfinite(vHatLeft)));

    if ekfStateFinite > 0.5 && ...
            pHatLeft(3) > cfg_visibilityZMin
        rhoHatRaw = 1/pHatLeft(3);
        rhoHatSafe = min( ...
            max(rhoHatRaw,cfg_rhoMin), ...
            cfg_rhoMax);
        ekfPredictionValid = 1;
    end

    Psym = 0.5*(P+P');
    traceP = trace(Psym);
    symmetryErrorP = norm(P-P','fro');
    eigenvaluesP = eig(Psym);
    minEigenvalueP = min(real(eigenvaluesP));
    return;
end

% 恒加速度状态模型
I3 = eye(3);
Z3 = zeros(3,3);
I9 = eye(9);
Ts = cfg_Ts;

F = [ ...
    I3, Ts*I3, 0.5*Ts*Ts*I3
    Z3, I3,    Ts*I3
    Z3, Z3,    I3
];

sigmaJerkSquared = cfg_sigmaJerk*cfg_sigmaJerk;

Q = sigmaJerkSquared * [ ...
    (Ts^5/20)*I3, (Ts^4/8)*I3, (Ts^3/6)*I3
    (Ts^4/8)*I3,  (Ts^3/3)*I3, (Ts^2/2)*I3
    (Ts^3/6)*I3,  (Ts^2/2)*I3, Ts*I3
];

% 预测
xPred = F*x;
PPred = F*P*F' + Q;
PPred = 0.5*(PPred+PPred');

pPredW = xPred(1:3);
pPredLeft = ...
    rotationCameraToWorld' * ...
    (pPredW-pCameraW);

predictionFinite = ...
    kinematicInputFinite && ...
    all(isfinite(xPred)) && ...
    all(isfinite(PPred(:))) && ...
    all(isfinite(pPredLeft));

ekfPredictionValid = double( ...
    predictionFinite && ...
    pPredLeft(3) > cfg_visibilityZMin);

% 默认采用预测结果
x = xPred;
P = PPred;

% 仅在新视觉消息到来时执行测量更新
measurementOK = ...
    measurementAvailable && ...
    ekfPredictionValid > 0.5;

if measurementOK
    Z = pPredLeft(3);
    rhoPred = 1/Z;
    xLeftPred = pPredLeft(1)/Z;
    yLeftPred = pPredLeft(2)/Z;

    h = [xLeftPred; yLeftPred; rhoPred];

    HLeft = [ ...
        rhoPred, 0,       -xLeftPred*rhoPred
        0,       rhoPred, -yLeftPred*rhoPred
        0,       0,       -rhoPred*rhoPred
    ];

    HWorld = HLeft*rotationCameraToWorld';
    H = [HWorld, zeros(3,3), zeros(3,3)];

    if all(isfinite(h)) && all(isfinite(H(:)))
        innovation = z-h;
        rhoInnovation = innovation(3);

        pixelVariance = ...
            cfg_pixelNoiseStd*cfg_pixelNoiseStd;
        fxLeft = max(fx(1),cfg_numericalEpsilon);
        fxRight = max(fx(2),cfg_numericalEpsilon);
        fyLeft = max(fy(1),cfg_numericalEpsilon);
        baseline = max(cfg_baseline,cfg_numericalEpsilon);

        varXLeft = pixelVariance/(fxLeft*fxLeft);
        varYLeft = pixelVariance/(fyLeft*fyLeft);
        covXLeftRho = ...
            pixelVariance/(baseline*fxLeft*fxLeft);
        varRho = pixelVariance/(baseline*baseline) * ...
            (1/(fxLeft*fxLeft)+1/(fxRight*fxRight));

        R = [ ...
            varXLeft,    0,        covXLeftRho
            0,           varYLeft, 0
            covXLeftRho, 0,        varRho
        ];

        R = R + cfg_ekfCovarianceJitter*eye(3);
        S = H*PPred*H' + R;

        innovationCovarianceValid = ...
            all(isfinite(S(:))) && ...
            rcond(S) > cfg_ekfSConditionMin;

        if innovationCovarianceValid
            K = (PPred*H')/S;
            xUpdated = xPred+K*innovation;
            A = I9-K*H;
            PUpdated = A*PPred*A'+K*R*K';
            PUpdated = 0.5*(PUpdated+PUpdated');

            if cfg_ekfCovarianceJitter > 0
                PUpdated = PUpdated + ...
                    cfg_ekfCovarianceJitter*I9;
            end

            updateFinite = ...
                all(isfinite(xUpdated)) && ...
                all(isfinite(PUpdated(:)));

            if updateFinite
                x = xUpdated;
                P = PUpdated;
                ekfMeasurementUpdated = 1;
            end
        end
    end
end

% 状态输出
pHatW = x(1:3);
vHatW = x(4:6);
aHatW = x(7:9);
pHatLeft = ...
    rotationCameraToWorld' * ...
    (pHatW-pCameraW);
vHatLeft = rotationCameraToWorld'*vHatW;

ekfStateFinite = double( ...
    all(isfinite(x)) && ...
    all(isfinite(P(:))) && ...
    all(isfinite(pHatLeft)) && ...
    all(isfinite(vHatLeft)));

if ekfStateFinite > 0.5 && ...
        pHatLeft(3) > cfg_visibilityZMin
    rhoHatRaw = 1/pHatLeft(3);
    rhoHatSafe = min( ...
        max(rhoHatRaw,cfg_rhoMin), ...
        cfg_rhoMax);
else
    rhoHatRaw = 0;
    rhoHatSafe = 0;
    ekfPredictionValid = 0;
end

innovationNorm = sqrt(innovation'*innovation);
Psym = 0.5*(P+P');
symmetryErrorP = norm(P-P','fro');
traceP = trace(Psym);
eigenvaluesP = eig(Psym);
minEigenvalueP = min(real(eigenvaluesP));

% 非有限状态自动复位并重新等待初始化
diagnosticsValid = ...
    ekfStateFinite > 0.5 && ...
    isfinite(traceP) && ...
    isfinite(minEigenvalueP) && ...
    isfinite(symmetryErrorP);

if ~diagnosticsValid
    x = ekfX0;
    P = ekfP0;
    initialized = false;

    pHatW = zeros(3,1);
    vHatW = zeros(3,1);
    aHatW = zeros(3,1);
    pHatLeft = zeros(3,1);
    vHatLeft = zeros(3,1);
    rhoHatRaw = 0;
    rhoHatSafe = 0;
    innovation = zeros(3,1);
    rhoInnovation = 0;
    innovationNorm = 0;
    traceP = trace(ekfP0);
    minEigenvalueP = 0;
    symmetryErrorP = 0;
    ekfPredictionValid = 0;
    ekfMeasurementUpdated = 0;
    ekfStateFinite = 0;
end
end

== matlab function stereo_ibvs_core_backup_20260724_005942/06_Estimated_Rho_Dynamics/Estimate Rho Dynamics ==
  data: normalizedFeatureMeasured input; rhoDotHat output; rhoHatSafe input; vHatCL input; vHatCR input; JL input; JR input; qDotAppliedDelayed input; cfg_numericalEpsilon input; rhoDynamicsValid output
function [rhoDotHat, rhoDynamicsValid] = fcn( ...
    normalizedFeatureMeasured, ...
    rhoHatSafe, ...
    vHatCL, ...
    vHatCR, ...
    JL, ...
    JR, ...
    qDotAppliedDelayed, cfg_numericalEpsilon)
%#codegen
% V2 Estimated Rho Dynamics
%
% 输入尺寸：
% normalizedFeatureMeasured : 4×1 [xL;yL;xR;yR]
% rhoHatSafe                : 1×1
% vHatCL                    : 3×1
% vHatCR                    : 3×1
% JL                        : 6×7
% JR                        : 6×7
% qDotAppliedDelayed        : 7×1
%
% 输出：
% rhoDotHat                 : 2×1
% rhoDynamicsValid          : 1×1

%% 固定尺寸输出
rhoDotHat = zeros(2,1);
rhoDynamicsValid = false;

features = reshape(normalizedFeatureMeasured,4,1);
velocityCL = reshape(vHatCL,3,1);
velocityCR = reshape(vHatCR,3,1);
qDotDelayed = reshape(qDotAppliedDelayed,7,1);

%% 输入有效性
inputValid = ...
    all(isfinite(features)) && ...
    isfinite(rhoHatSafe) && ...
    all(isfinite(velocityCL)) && ...
    all(isfinite(velocityCR)) && ...
    all(isfinite(JL(:))) && ...
    all(isfinite(JR(:))) && ...
    all(isfinite(qDotDelayed)) && ...
    isfinite(cfg_numericalEpsilon) && ...
    cfg_numericalEpsilon > 0 && ...
    rhoHatSafe > cfg_numericalEpsilon;

if ~inputValid
    return;
end

rho = max(rhoHatSafe, cfg_numericalEpsilon);

%% 左相机
xL = features(1);
yL = features(2);

LrhoL = [
    0, 0, rho*rho, ...
    rho*yL, -rho*xL, 0
];

Hrho = [0, 0, -rho*rho];

cameraVelocityLeft = JL * qDotDelayed;

rhoDotHat(1) = ...
    LrhoL * cameraVelocityLeft + ...
    Hrho * velocityCL;

%% 右相机
xR = features(3);
yR = features(4);

LrhoR = [
    0, 0, rho*rho, ...
    rho*yR, -rho*xR, 0
];

cameraVelocityRight = JR * qDotDelayed;

rhoDotHat(2) = ...
    LrhoR * cameraVelocityRight + ...
    Hrho * velocityCR;

%% 最终数值保护
if all(isfinite(rhoDotHat))
    rhoDynamicsValid = true;
else
    rhoDotHat = zeros(2,1);
    rhoDynamicsValid = false;
end
end

== matlab function stereo_ibvs_core_backup_20260724_005942/07_Arm_Priority_Controller/Final Arm Priority Controller ==
  data: q input; qDotCmd output; cLMeasured input; rhoHatL input; vHatLeft input; JL input; cLd input; rhoD input; validLeft input; ekfPredictionValid input; centerEnable input; depthEnable input; armEnable input; depthTaskWeight input; cfg_numericalEpsilon input; cfg_robustEnable input; cfg_betaC input; cfg_epsilonC input; cfg_Kc input; cfg_lambdaC input; cfg_betaRho input; cfg_epsilonRho input; cfg_kRho input; cfg_lambdaRho input; cfg_nullspaceEnable input; cfg_kNull input; cfg_qMid input; cfg_leftOnlyCenterControlEnable input; centerError output; depthError output; rcondJc output; rcondArho output; qDotCenter output; qDotDepthRaw output; qDotDepthWeighted output; qDotNullUsed output
function [qDotCmd,centerError,depthError,rcondJc,rcondArho,qDotCenter,qDotDepthRaw,qDotDepthWeighted,qDotNullUsed] = ...
    fcn(q,cLMeasured,rhoHatL,vHatLeft,JL,cLd,rhoD,validLeft,ekfPredictionValid,centerEnable,depthEnable,armEnable,depthTaskWeight, ...
    cfg_numericalEpsilon,cfg_robustEnable,cfg_betaC,cfg_epsilonC,cfg_Kc,cfg_lambdaC,cfg_betaRho,cfg_epsilonRho,cfg_kRho,cfg_lambdaRho,cfg_nullspaceEnable,cfg_kNull,cfg_qMid,cfg_leftOnlyCenterControlEnable)
%#codegen
% 代码作用：
% 左相机归一化中心为主任务，逆深度为次任务。
% 支持目标速度前馈、鲁棒项、阻尼伪逆和关节中位零空间任务。

qDotCmd = zeros(7,1);
centerError = zeros(2,1);
depthError = 0;
rcondJc = 0;
rcondArho = 0;
qDotCenter = zeros(7,1);
qDotDepthRaw = zeros(7,1);
qDotDepthWeighted = zeros(7,1);
qDotNullUsed = zeros(7,1);

x = cLMeasured(1);
y = cLMeasured(2);
rho = rhoD;
vFeed = zeros(3,1);

if ekfPredictionValid > 0.5 && ...
        isfinite(rhoHatL) && rhoHatL > 0 && ...
        all(isfinite(vHatLeft))
    rho = max(rhoHatL,cfg_numericalEpsilon);
    vFeed = vHatLeft;
end

centerError = [x;y] - cLd;
depthError = rho - rhoD;

Lc = [
    -rho, 0, x*rho, x*y, -(1+x*x), y
    0, -rho, y*rho, 1+y*y, -x*y, -x
];

Hc = rho*[1 0 -x;0 1 -y];
bhatC = Hc*vFeed;
Jc = Lc*JL;

rc = zeros(2,1);
if cfg_robustEnable > 0.5
    rc = cfg_betaC*centerError / ...
        (sqrt(centerError'*centerError)+cfg_epsilonC);
end

nuC = -cfg_Kc*centerError - bhatC - rc;
Gc = Jc*Jc' + cfg_lambdaC^2*eye(2);
JcSharp = Jc'/Gc;
qC = JcSharp*nuC;
Nc = eye(7)-JcSharp*Jc;
rcondJc = det(Gc) / ...
    (trace(Gc)*trace(Gc)+cfg_numericalEpsilon);
qDotCenter = qC;

Lrho = [0 0 rho*rho rho*y -rho*x 0];
Hrho = [0 0 -rho*rho];
Jrho = Lrho*JL;
bhatRho = Hrho*vFeed;

rr = 0;
if cfg_robustEnable > 0.5
    rr = cfg_betaRho*depthError / ...
        (abs(depthError)+cfg_epsilonRho);
end

nuRho = -cfg_kRho*depthError-bhatRho-rr;
A = Jrho*Nc;
denom = A*A'+cfg_lambdaRho^2;
rcondArho = denom/(1+denom);

w = min(max(depthTaskWeight,0),1) * ...
    double(ekfPredictionValid > 0.5);
qDotDepthRaw = Nc*A'*((nuRho-Jrho*qC)/denom);
qDotDepthWeighted = w*qDotDepthRaw;

qDot0 = zeros(7,1);
if cfg_nullspaceEnable > 0.5
    qDot0 = -cfg_kNull*(q-cfg_qMid);
end

ArhoDagger = A'/denom;
NcRho = Nc*(eye(7)-ArhoDagger*A);
Nnull = (1-w)*Nc+w*NcRho;
qDotNullUsed = Nnull*qDot0;

if centerEnable > 0.5
    qDotCmd = qDotCenter+qDotNullUsed;
end

if centerEnable > 0.5 && depthEnable > 0.5
    qDotCmd = qDotCenter+qDotDepthWeighted+qDotNullUsed;
end

if centerEnable <= 0.5 && depthEnable > 0.5
    d = Jrho*Jrho'+cfg_lambdaRho^2;
    qDotDepthRaw = Jrho'*(nuRho/d);
    qDotDepthWeighted = w*qDotDepthRaw;
    qDotCenter = zeros(7,1);
    qDotNullUsed = zeros(7,1);
    qDotCmd = qDotDepthWeighted;
end

centerAllowed = validLeft > 0.5 && ...
    cfg_leftOnlyCenterControlEnable > 0.5;

if ~centerAllowed || armEnable <= 0.5
    qDotCmd = zeros(7,1);
    qDotCenter = zeros(7,1);
    qDotDepthWeighted = zeros(7,1);
    qDotNullUsed = zeros(7,1);
end

if any(~isfinite(qDotCmd))
    qDotCmd = zeros(7,1);
end
end
